simulink model "airtrim"  (R2023b)
settings: Solver=ode45  StartTime=0.0  StopTime=10.0  RelTol=1e-3  EnableMultiTasking=on
libraries: airlib x1
settings Model: Creator=Elisa  LastModifiedBy=Elisa
settings DataIOCC: ExternalInput=[0 1 0 0 0 0 0 0 0 0 6.7015280237240514e-017]  InitialState=[100;0.33384643595852526;0;0;0;0;0;0.33384643595852531;0;0;0;60]  LoadExternalInput=on  LoadInitialState=on  SaveFormat=Array  SignalLoggingSaveFormat=ModelDataLogs  ReturnWorkspaceOutputs=off
settings OptimizationCC: BlockReduction=off  BooleanDataType=off
settings DebuggingCC: SaveWithParameterizedLinksMsg=none  UnderspecifiedInitializationDetection=Classic  MergeDetectMultiDrivingBlocksExec=none  SignalResolutionControl=TryResolveAllWithWarning  MultiTaskDSMMsg=warning  MultiTaskCondExecSysMsg=none  UnconnectedInputMsg=warning  UnconnectedOutputMsg=warning  UnconnectedLineMsg=warning
settings HardwareCC: TargetUnknown=on
settings ModelReferenceCC: PropagateSignalLabelsOutOfModel=off
settings GRTTargetCC: CombineOutputUpdateFcns=off  GRTInterface=on

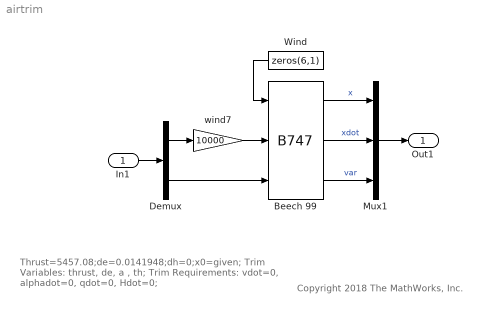
== system airtrim ==
  note: Thrust=5457.08;de=0.0141948;dh=0;x0=given;
      | Trim Variables: thrust, de, a , th;
      | Trim Requirements: vdot=0, alphadot=0, qdot=0, Hdot=0;
  note: Copyright 2018 The MathWorks, Inc.
  In1 : Inport
  " Beech 99 " : airlib/B747  GM1="[1.9812   14.0208  26.0129  13673  20538  31246   0  2169.3  0   3175.2]"  CD_wind="[0.027   0.131  0  0  0]"  CL_wind="[0.201   5.48    8.1   0.6   0]"  Cm_body="[0.05  -1.89  -34.0   -2.0   0]"  CY_body="[0  -0.59  -0.19  0.39  0.0  0.148]"  Cl_body="[0    -0.13  -0.5  0.14  -0.156  0.0109]"  Cn_body="[0    0.08   0.0109  -0.197  0.0012  -0.0772]"  x0="[100  -0.00393591 0   0 0 0   0 -0.00393591 0   0 0 60]"
      settings: SourceProductName=Aircraft Library
  Demux : Demux  Outputs=[6 4]
      settings: DisplayOption=none
  Mux1 : Mux  Inputs=[12 12 12]
  Wind : Constant  Value=zeros(6,1)
  wind7 : Gain  Gain=10000  SaturateOnIntegerOverflow=on  OutDataTypeStr=Inherit: Same as input  ParamDataTypeStr=Inherit: Same as input
  Out1 : Outport
  wires:
  Demux/1 -> wind7/1
  In1/1 -> Demux/1
  Mux1/1 -> Out1/1
  Wind/1 -> " Beech 99 "/1
  wind7/1 -> " Beech 99 "/2
  Demux/2 -> " Beech 99 "/3
  " Beech 99 "/1 -> Mux1/1  "x"
  " Beech 99 "/2 -> Mux1/2  "xdot"
  " Beech 99 "/3 -> Mux1/3  "var"
